simulink model "FeedbackLinearizedArm"  (R2014b)
settings: Solver=ode3  StartTime=0.0  StopTime=10.0  FixedStep=0.01  RelTol=1e-3
values from neighbouring files (symbols this model uses):
  G = [zeros(2); eye(2)]    [FeedbackTestScript.m]    (also in Hanoi_SlidingControl_GUI.m = [zeros(2,2);eye(2)])
  Kd = eye(2)*14    [FeedbackTestScript.m]    (also in Hanoi_SlidingControl_GUI.m = eye(2)*74)
  Kp = eye(2)*316    [FeedbackTestScript.m]    (also in Hanoi_SlidingControl_GUI.m = eye(2)*2236.1)
  P = lyap(F', eye(4))    [FeedbackTestScript.m]    (also in Hanoi_SlidingControl_GUI.m = eye(4))
  U = eye(2)    [FeedbackTestScript.m]    (also in Hanoi_SlidingControl_GUI.m = str2double(get(handles.SC_GainEntry,'String')))
settings Model: Creator=lpark_000  LastModifiedBy=gkhadge
settings DataIOCC: LimitDataPoints=off

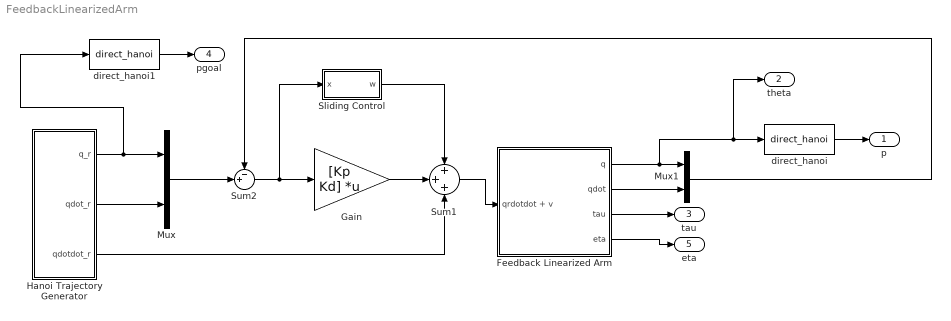
== system FeedbackLinearizedArm ==
  Feedback Linearized Arm : Subsystem
  Gain : Gain  Gain=[Kp Kd]  Multiplication=Matrix(K*u)
  Hanoi Trajectory Generator : Subsystem
  Mux : Mux  Inputs=2
  Mux1 : Mux  Inputs=2
  Sliding Control : Subsystem
  Sum1 : Sum  Inputs=+++
  Sum2 : Sum  Inputs=-+|
  direct_hanoi : MATLABFcn  MATLABFcn=direct_hanoi
  direct_hanoi1 : MATLABFcn  MATLABFcn=direct_hanoi
  p : Outport
  theta : Outport  Port=2
  tau : Outport  Port=3
  pgoal : Outport  Port=4
  eta : Outport  Port=5
  wires:
  Hanoi Trajectory Generator/2(qdot_r) -> Mux/2
  Sum1/1 -> Feedback Linearized Arm/1(qrdotdot + v)
  Feedback Linearized Arm/1(q) -> theta/1, direct_hanoi/1, Mux1/1
  Feedback Linearized Arm/2(qdot) -> Mux1/2
  Sum2/1 -> Sliding Control/1(x), Gain/1
  Mux/1 -> Sum2/2
  Mux1/1 -> Sum2/1
  direct_hanoi/1 -> p/1
  Gain/1 -> Sum1/2
  Hanoi Trajectory Generator/3(qdotdot_r) -> Sum1/3
  Sliding Control/1(w) -> Sum1/1
  Feedback Linearized Arm/3(tau) -> tau/1
  Hanoi Trajectory Generator/1(q_r) -> direct_hanoi1/1, Mux/1
  direct_hanoi1/1 -> pgoal/1
  Feedback Linearized Arm/4(eta) -> eta/1

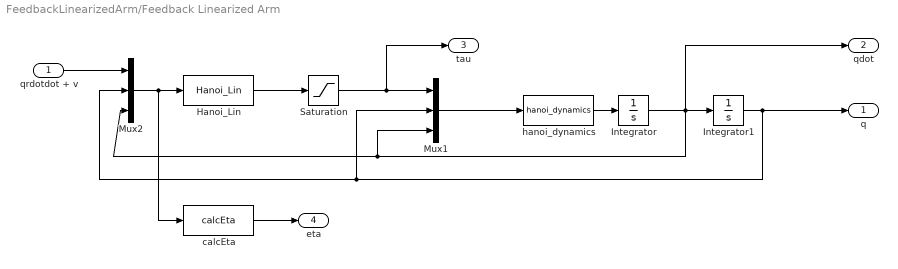
== system FeedbackLinearizedArm/Feedback Linearized Arm ==
  qrdotdot + v : Inport
  Hanoi_Lin : MATLABFcn  MATLABFcn=Hanoi_Lin
  Integrator : Integrator  InitialCondition=[0; 0]
  Integrator1 : Integrator  InitialCondition=[pi/2; -pi/2]
  Mux1 : Mux  Inputs=3
  Mux2 : Mux  Inputs=3
  Saturation : Saturate  UpperLimit=3  LowerLimit=-3
  calcEta : MATLABFcn  MATLABFcn=calcEta
  hanoi_dynamics : MATLABFcn  MATLABFcn=hanoi_dynamics
  q : Outport
  qdot : Outport  Port=2
  tau : Outport  Port=3
  eta : Outport  Port=4
  wires:
  Mux1/1 -> hanoi_dynamics/1
  Integrator/1 -> Integrator1/1, qdot/1, Mux2/3, Mux1/3
  hanoi_dynamics/1 -> Integrator/1
  Integrator1/1 -> q/1, Mux2/2, Mux1/2
  qrdotdot + v/1 -> Mux2/1
  Mux2/1 -> calcEta/1, Hanoi_Lin/1
  Hanoi_Lin/1 -> Saturation/1
  Saturation/1 -> tau/1, Mux1/1
  calcEta/1 -> eta/1

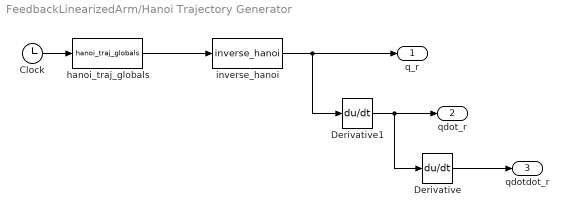
== system FeedbackLinearizedArm/Hanoi Trajectory Generator ==
  Clock : Clock
  Derivative : Derivative
  Derivative1 : Derivative
  hanoi_traj_globals : MATLABFcn  MATLABFcn=hanoi_traj_globals
  inverse_hanoi : MATLABFcn  MATLABFcn=inverse_hanoi
  q_r : Outport
  qdot_r : Outport  Port=2
  qdotdot_r : Outport  Port=3
  wires:
  Clock/1 -> hanoi_traj_globals/1
  inverse_hanoi/1 -> q_r/1, Derivative1/1
  Derivative1/1 -> qdot_r/1, Derivative/1
  Derivative/1 -> qdotdot_r/1
  hanoi_traj_globals/1 -> inverse_hanoi/1

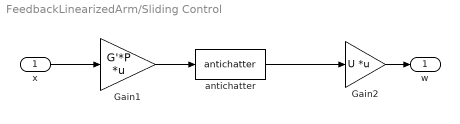
== system FeedbackLinearizedArm/Sliding Control ==
  x : Inport
  Gain1 : Gain  Gain=G'*P  Multiplication=Matrix(K*u)
  Gain2 : Gain  Gain=U  Multiplication=Matrix(K*u)
  antichatter : MATLABFcn  MATLABFcn=antichatter
  w : Outport
  wires:
  Gain2/1 -> w/1
  x/1 -> Gain1/1
  Gain1/1 -> antichatter/1
  antichatter/1 -> Gain2/1
